simulink model "picontroller"  (R2020b)
settings: Solver=VariableStepAuto  StartTime=0.0  StopTime=120  MaxStep=0.01  RelTol=1e-3
values from neighbouring files (symbols this model uses):
  kd = 0.18    [data_q3.sldd]
  ki = 90.0    [data_q3.sldd]
  kp = 550.0    [data_q3.sldd]
settings Model: DataDictionary=data_q3.sldd  Creator=Ravi  LastModifiedBy=Ravi
settings DataIOCC: SaveOutput=off  SaveTime=off

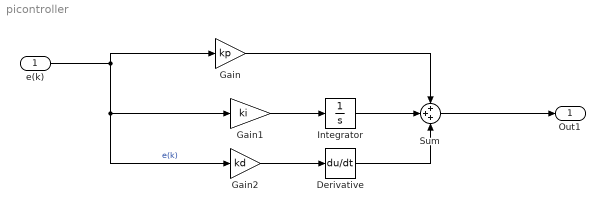
== system picontroller ==
  e(k) : Inport  OutDataTypeStr=double  PortDimensions=1  SampleTime=0
  Derivative : Derivative
  Gain : Gain  Gain=kp
  Gain1 : Gain  Gain=ki
  Gain2 : Gain  Gain=kd
  Integrator : Integrator
  Sum : Sum  Inputs=+++
  Out1 : Outport  OutDataTypeStr=double  PortDimensions=1  SampleTime=0
  wires:
  Gain1/1 -> Integrator/1
  e(k)/1 -> Gain/1, Gain1/1, Gain2/1  "e(k)"
  Integrator/1 -> Sum/2
  Gain2/1 -> Derivative/1
  Derivative/1 -> Sum/3
  Gain/1 -> Sum/1
  Sum/1 -> Out1/1
